simulink model "hdv_hydroelectropowertrain_model"  (R2023b)
settings: Solver=ode1be  StartTime=0.0  StopTime=simulation_length  FixedStep=tsample  MaxStep=tsample
values from neighbouring files (symbols this model uses):
  alpha = 35    [init_model.m]
  Apump = [0 1; 0 0]    [init_model.m]
  available_torque = torque_base+torque_friction_base    [init_model.m]
  Bpump = [0 1]'    [init_model.m]
  btheta_shaft = 2e2    (= 200)    [init_model.m]
  C1 = 10    [init_model.m]
  consumption = [consumption_1, consumption_2, consumption_3, consumption_4,          consumption_5, consumption_6, consumption_7, consumption_8,          consumption_9, consumption_10, consumption_11, consumption_12,          consumption_13, consumption_14, consumption_15, consumption_16          ]    [ic_engine_data.m]
  Cpump = [k 0]    [init_model.m]
  dp_lim = 400    [init_model.m]
  E0 = 3.685    [init_model.m]
  E1 = 0.2156    [init_model.m]
  E2 = 0    [init_model.m]
  E3 = 0    [init_model.m]
  E_1 = -1.031    [init_model.m]
  Elog = -0.05    [init_model.m]
  eta_v_m = 0.98    [init_model.m]
  eta_v_p = 0.97    [init_model.m]
  ki_dp_comp = 1/dp_lim    (= 0.0025)    [init_model.m]
  ki_te_comp = 2/te_lim    [init_model.m]
  kp_ctrl_m = 1    [init_model.m]
  kp_dp_comp = 0.5/dp_lim    (= 0.00125)    [init_model.m]
  kp_te_comp = 1/te_lim    [init_model.m]
  Kpump = acker(Apump,Bpump,poles)    [init_model.m]
  load_blade_enable = 0    [init_model.m]
  Lpump = acker(Apump',Cpump',pole_so)'    [init_model.m]
  M = 125    [init_model.m]
  Ncell = 185    [init_model.m]
  Npump = -1/(Cpump*inv(Apump-Bpump*Kpump)*Bpump)    [init_model.m]
  omega_e_rpm_ref = 1700    [init_model.m]
  omega_l_max_rpm = omega_l_max/(2*pi)*60    (= 50.3075969543)    [init_model.m]
  q1Kalman = tsample^2*1e-2    (= 1e-08)    [init_model.m]
  q2Kalman = tsample^1*1e-1    (= 0.0001)    [init_model.m]
  q3Kalman = 0    [init_model.m]
  Qhr = 400    [init_model.m]
  R0 = 0.015    [init_model.m]
  R1 = 0.015    [init_model.m]
  R_tg = 1.16/2    (= 0.58)    [init_model.m]
  rKalman = 1    [init_model.m]
  rpm_base = [620 700 800 900 1000 1100 1200 1300 1400 1500 1600 1700 1800      1900 2000 2100]    [ic_engine_data.m]
  rpm_consumption = rpm_base    [ic_engine_data.m]
  simulation_length = 245    [init_model.m]
  tau_load = 75e3    (= 75000)    [init_model.m]
  tau_load_max = 1600*41.4    (= 66240)    [init_model.m]
  Tc = tsample    (= 0.001)    [init_model.m]
  torque_base = [max(torque_16_data) max(torque_15_data) max(torque_14_data)      max(torque_13_data) max(torque_12_data) max(torque_11_data)      max(torque_10_data) max(torque_9_data) max(torque_8_data)      max(torque_7_data) max(torque_6_data) max(torque_5_data)      max(torque_4_data) max(torque_3_data) max(torque_2_data)      max(torque_1_data)]    [ic_engine_data.m]
  torque_consumption = torque_reference    [ic_engine_data.m]
  torque_friction_base = -(rpm_base./60*2*pi)*0.25-(rpm_base./60*2*pi).^2*5.2e-4    [ic_engine_data.m]
  tsample = 1e-3    (= 0.001)    [init_model.m]
  v_track1_ref = 8    [init_model.m]
  v_track2_ref = 8    [init_model.m]
  valve_mmorifice_max = 2.75    [init_model.m]
  xv_m_max = 1.2    [init_model.m]
undefined symbols (not defined in the file or in its folder): magnitude
libraries: fl_lib x381, nesl_utility x162, linear_swashplate_ctrl_lib x8, flexshaft_lib x5, bichamber_piston_lib x5, variable_displacement_motor_lib x4, variable_displacement_pump_lib x4, fixed_displacement_pump_lib x4, relief_valve_lib x4, inverse_shuttle_valve_lib x4, hydrostatic_threeway_valve_bichamber_piston_lib x4, hydrostatic_fourway_valve_bichamber_piston_lib x4
(part 3 of 9)

== system hdv_hydroelectropowertrain_model/PR776_powertrain/constant_pressure_source/Pressure controlled pump1 ==
  Hydraulic Flow Rate Sensor : fl_lib/Hydraulic/Hydraulic Sensors/Hydraulic Flow Rate Sensor
  Hydraulic Pressure Sensor : fl_lib/Hydraulic/Hydraulic Sensors/Hydraulic Pressure Sensor
  Hydraulic Reference : fl_lib/Hydraulic/Hydraulic Elements/Hydraulic Reference
  PS-Simulink Converter : nesl_utility/PS-Simulink Converter  PhysicalDomain=network_engine_domain  SubClassName=ps_output  LeftPortType=input  RightPortType=output  PseudoPeriodic=off  Frequencies=[]  VectorFormat=1-D array  Unit=bar  AffineConversion=on
  PS-Simulink Converter1 : nesl_utility/PS-Simulink Converter  PhysicalDomain=network_engine_domain  SubClassName=ps_output  LeftPortType=input  RightPortType=output  PseudoPeriodic=off  Frequencies=[]  VectorFormat=1-D array  Unit=l/min  AffineConversion=on
  PS-Simulink Converter{2..5} (4 alike) : nesl_utility/PS-Simulink Converter  PhysicalDomain=network_engine_domain  SubClassName=ps_output  LeftPortType=input  RightPortType=output  PseudoPeriodic=off  Frequencies=[]  VectorFormat=1-D array  Unit=1  AffineConversion=off
  Pressure controlled pump : pressure_controlled_pump_lib/Pressure controlled pump  Vd_nom=62.3*4 cm^3/rev  pnom=250 bar  b=0.1 N*m/(rad/s)  inertia_pump=0.027 kg*m^2  vd_lim_max=0.98  vd_lim_min=0  p_set=258 bar  p_reg=8 bar  x_rv_max=12 mm  kpc=2  kic=40 1/s  te_specify=off  te_priority=None  te=0 N*m  te_nominal_specify=off  te_nominal_unit=N*m  te_nominal_value=1  qA_specify=off  qA_priority=None  qA=0 m^3/s  qA_nominal_specify=off  qA_nominal_unit=m^3/s  qA_nominal_value=1  qB_specify=off  qB_priority=None  qB=0 m^3/s  qB_nominal_specify=off  qB_nominal_unit=m^3/s  qB_nominal_value=1  qd_specify=off  qd_priority=None  qd=0 m^3/s  qd_nominal_specify=off  qd_nominal_unit=m^3/s  qd_nominal_value=1  dp_specify=off  dp_priority=None  dp=0 Pa  dp_nominal_specify=off  dp_nominal_unit=Pa  dp_nominal_value=1  vd_specify=off  vd_priority=None  vd=0  vd_nominal_specify=off  vd_nominal_unit=1  vd_nominal_value=1  vd_i_specify=off  vd_i_priority=None  vd_i=0  vd_i_nominal_specify=off  vd_i_nominal_unit=1  vd_i_nominal_value=1  we_specify=off  we_priority=None  we=0 rad/s  we_nominal_specify=off  we_nominal_unit=rad/s  we_nominal_value=1
      settings: InternalSimscapePortConfiguration="{\"Bottom\":[],\"Left\":[{\"id\":\"cW\",\"label\":\"cW\",\"type\":\"foundation.mechanical.rotational.rotational\"},{\"id\":\"dp_ref\",\"label\":\"Pressure set-point\",\"type\":\"input\"}],\"Right\":[{\"id\":\"cA\",\"label\":\"cA\",\"type\":\"foundation.hydraulic.hydraulic\"},{\"id\":\"cB\",\"label\":\"cB\",\"type\":\"foundation.hydraulic.hydraulic\"},{\"id\":\"qleak\",\"label\":\"qleak\",\"type\":\"output\"},{\"id\":\"taup\",\"label\":\"taup\",\"type\":\"output\"},{\"id\":\"vdi\",\"label\":\"vdi\",\"type\":\"output\"},{\"id\":\"pflow\",\"label\":\"pflow\",\"type\":\"output\"}],\"Top\":[]}"
  flow : Scope
  leak/ptorque : Scope  NumInputPorts=3
  pressure : Scope
  pump_flow : Scope
  pS : PMIOPort  Side=Right
  shaft : PMIOPort  Port=2  Side=Left
  pT : PMIOPort  Port=3  Side=Right
  wires:
  PS-Simulink Converter1/1 -> flow/1
  PS-Simulink Converter4/1 -> leak/ptorque/3  "vd"
  PS-Simulink Converter3/1 -> leak/ptorque/2  "torque"
  PS-Simulink Converter5/1 -> pump_flow/1
  PS-Simulink Converter2/1 -> leak/ptorque/1  "leak"
  PS-Simulink Converter/1 -> pressure/1
  connections:
  shaft/RConn1 -- Pressure controlled pump/LConn1
  Pressure controlled pump/RConn4 -- PS-Simulink Converter3/LConn1
  Pressure controlled pump/RConn3 -- PS-Simulink Converter2/LConn1
  Hydraulic Flow Rate Sensor/RConn1 -- PS-Simulink Converter1/LConn1
  Hydraulic Pressure Sensor/LConn1 -- pS/RConn1 -- Hydraulic Flow Rate Sensor/RConn2
  Hydraulic Reference/LConn1 -- Pressure controlled pump/RConn2 -- pT/RConn1 -- Hydraulic Pressure Sensor/RConn1
  Pressure controlled pump/RConn1 -- Hydraulic Flow Rate Sensor/LConn1
  Pressure controlled pump/RConn5 -- PS-Simulink Converter4/LConn1
  Pressure controlled pump/RConn6 -- PS-Simulink Converter5/LConn1
  PS-Simulink Converter/LConn1 -- Hydraulic Pressure Sensor/RConn2

== system hdv_hydroelectropowertrain_model/PR776_powertrain/electrical_main_drive_train/LithiumIonBattery ==
  Bus Creator : BusCreator  Inputs=4
  Current Sensor : fl_lib/Electrical/Electrical Sensors/Current Sensor
  Current Sensor1 : fl_lib/Electrical/Electrical Sensors/Current Sensor
  Electrical Reference1 : fl_lib/Electrical/Electrical Elements/Electrical Reference
  PS-Simulink Converter1 : nesl_utility/PS-Simulink Converter  PhysicalDomain=network_engine_domain  SubClassName=ps_output  LeftPortType=input  RightPortType=output  PseudoPeriodic=off  Frequencies=[]  VectorFormat=1-D array  Unit=1  AffineConversion=off
  PS-Simulink Converter4 : nesl_utility/PS-Simulink Converter  PhysicalDomain=network_engine_domain  SubClassName=ps_output  LeftPortType=input  RightPortType=output  PseudoPeriodic=off  Frequencies=[]  VectorFormat=1-D array  Unit=1  AffineConversion=off
  PS-Simulink Converter5 : nesl_utility/PS-Simulink Converter  PhysicalDomain=network_engine_domain  SubClassName=ps_output  LeftPortType=input  RightPortType=output  PseudoPeriodic=off  Frequencies=[]  VectorFormat=1-D array  Unit=V  AffineConversion=on
  Resistor1 : fl_lib/Electrical/Electrical Elements/Resistor  R=1e4 Ohm  i_specify=off  i_priority=None  i=0 A  i_nominal_specify=off  i_nominal_unit=A  i_nominal_value=1  v_specify=off  v_priority=None  v=0 V  v_nominal_specify=off  v_nominal_unit=V  v_nominal_value=1
  Resistor2 : fl_lib/Electrical/Electrical Elements/Resistor  R=1e4 Ohm  i_specify=off  i_priority=None  i=0 A  i_nominal_specify=off  i_nominal_unit=A  i_nominal_value=1  v_specify=off  v_priority=None  v=0 V  v_nominal_specify=off  v_nominal_unit=V  v_nominal_value=1
  Unit Delay5 : UnitDelay  SampleTime=tsample  HasFrameUpgradeWarning=on
  Voltage Sensor : fl_lib/Electrical/Electrical Sensors/Voltage Sensor
  lithium ion cell analytical ocv : Subsystem
  Uout+ : PMIOPort  Side=Right
  Uout- : PMIOPort  Port=2  Side=Right
  Uin+ : PMIOPort  Port=3  Side=Left
  Uin- : PMIOPort  Port=4  Side=Left
  lithiumIonBattery_Data : Outport
  tag scope: vout_battery=global
  wires:
  PS-Simulink Converter5/1 -> Unit Delay5/1
  PS-Simulink Converter4/1 -> [iout_battery]  "i batt"
  Unit Delay5/1 -> [vout_battery]
  Bus Creator/1 -> lithiumIonBattery_Data/1
  [iout_battery] -> Bus Creator/1  "Iout_battery"
  [vout_battery] -> Bus Creator/2  "Vout_battery"
  [soc_battery] -> Bus Creator/3  "soc_battery"
  PS-Simulink Converter1/1 -> [iin_battery]  "i batt"
  [iin_battery] -> Bus Creator/4  "iin_battery"
  connections:
  Current Sensor/RConn1 -- PS-Simulink Converter4/LConn1
  Current Sensor/RConn2 -- Voltage Sensor/LConn1 -- Resistor2/LConn1 -- Uout+/RConn1
  Voltage Sensor/RConn1 -- PS-Simulink Converter5/LConn1
  Voltage Sensor/RConn2 -- Resistor1/RConn1 -- Uin-/RConn1 -- Electrical Reference1/LConn1 -- lithium ion cell analytical ocv/RConn2 -- Resistor2/RConn1 -- Uout-/RConn1
  lithium ion cell analytical ocv/RConn1 -- Current Sensor1/RConn2 -- Current Sensor/LConn1
  Current Sensor1/RConn1 -- PS-Simulink Converter1/LConn1
  Uin+/RConn1 -- Resistor1/LConn1 -- Current Sensor1/LConn1

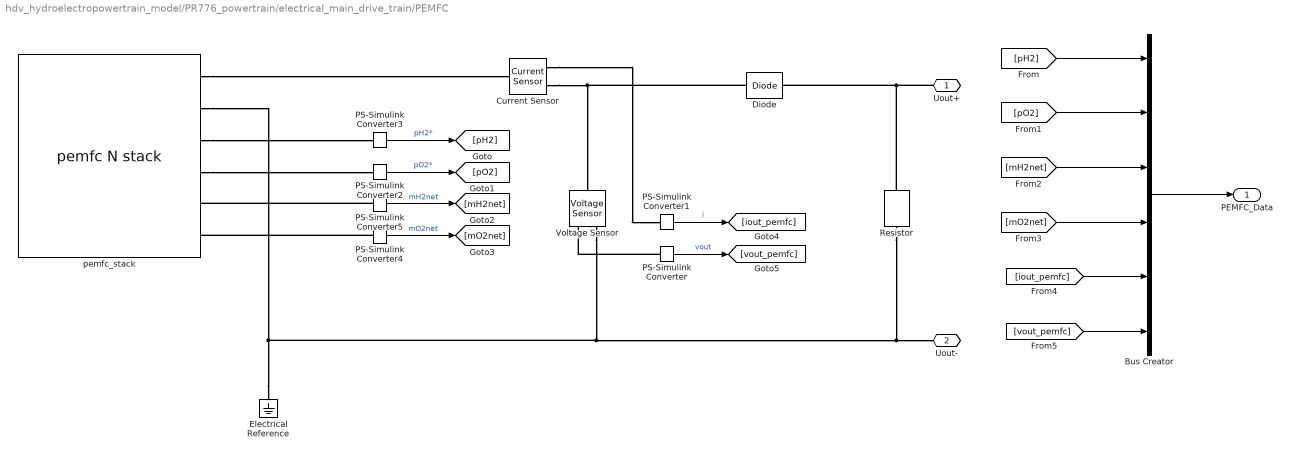
== system hdv_hydroelectropowertrain_model/PR776_powertrain/electrical_main_drive_train/PEMFC ==
  Bus Creator : BusCreator  Inputs=6
  Current Sensor : fl_lib/Electrical/Electrical Sensors/Current Sensor
  Diode : ee_lib/Semiconductors & Converters/Diode  ModelType=ee.enum.diode.modelType.pwl  TableType=ee.enum.diode.tableType.IfMat  IfMat=[.07, .12, .19, 1.75, 4.24, 7.32, 11.2; .16, .3, .72, 2.14, 5.02, 8.35, 13.12] A  VfMat=[.9, 1.15, 1.25, 1.5, 1.75, 2.17, 2.6, 2.85; .58, .68, .75, 1.1, 1.38, 1.77, 2.27, 2.7] V  TjVec=[25, 125] degC  VfVec=[.5, .7, .9, 1.3, 1.7, 2.1, 2.5] V  IfVec=[.1, .2, .5, 1, 2, 4, 7, 10] A  Vf=0.6 V  Ron=0.3 Ohm  Goff=1e-8 S  prmExp=ee.enum.diode.expParam.useTwo  I12=[.0137, .545] A  V12=[.6, .7] V  RS=0 Ohm  Tmeas=25 degC  IS=1e-12 A  ec=1  I1=0.0137 A  V1=0.6 V  N_series=1  N_parallel=1  ZenerEnable=false  Rz=0.3 Ohm  BV=inf V  C_param=ee.enum.diode.capParam.fixed  CJ=5 pF  CJ0=5 pF  Vvec=[.1, 10, 100] V  Cvec=[3.5, 1, .4] pF  VJ=1 V  Mgrad=0.5  FC=0.5  Q_param=ee.enum.diode.recoveryParam.off  iRM=-7.15 A  iF=4 A  didt=-750 A/us  trr_factor=3  trr=115 ns  Qrr=1500 s*uA  Vr=-600 V  Ls=150 nH  Erec=0.03 J  TT=50 ns  tau=100 ns  T_param=ee.enum.diode.temperatureParam.off  Tdevice=25 degC  I1_T2=0.245 A  V1_T2=0.5 V  IS_T2=1.25e-7 A  Tmeas2=125 degC  XTI_param=ee.enum.diode.xtiParam.pn  XTI=3  EG_param=ee.enum.diode.egapParam.material_si  EG=1.11 eV  dBVdT=0 V/K  enable_faults=ee.enum.enable.no  fault_action=simscape.enum.assert.action.none  fault_types=ee.enum.diode.faults.open  tau_fault=1e-3 s  IfMat_faulted=[.07, .12, .19, 1.75, 4.24, 7.32, 11.2; .16, .3, .72, 2.14, 4.02, 6.35, 9.12] A  VfMat_faulted=[.9, 1.15, 1.25, 1.5, 1.75, 2.17, 2.6, 2.85; .58, .68, .75, 1.1, 1.38, 1.77, 2.27, 2.7] V  VfVec_faulted=[.5, .7, .9, 1.3, 1.7, 2.1, 2.5] V  IfVec_faulted=[.1, .2, .5, 1, 2, 4, 7, 10] A  Ropen_faulted=1000 Ohm  Gshort_faulted=1000 1/Ohm  Vf_faulted=0.6 V  Ron_faulted=0.3 Ohm  Goff_faulted=1e-8 S  I12_faulted=[.0137, .545] A  V12_faulted=[.6, .7] V  IS_faulted=1e-12 A  ec_faulted=1  I1_faulted=0.0137 A  V1_faulted=0.6 V  RS_faulted=0 Ohm  Rz_faulted=0.3 Ohm  BV_faulted=inf V  Cscale_faulted=100  fault_trigger=ee.enum.faults.faultTrigger.temporal  t_fault=inf s  max_permissible_voltage=inf V  n_fail_on_voltage=1  max_permissible_current=inf A  t_fail_on_current=1 s  max_permissible_dVdt=inf V/s  enable_fault_input=simscape.enum.onoff.off  i_specify=off  i_priority=None  i=0 A  i_nominal_specify=off  i_nominal_unit=A  i_nominal_value=1  v_specify=off  v_priority=None  v=0 V  v_nominal_specify=off  v_nominal_unit=V  v_nominal_value=1  v_capacitor_specify=off  v_capacitor_priority=None  v_capacitor=0 V  v_capacitor_nominal_specify=off  v_capacitor_nominal_unit=V  v_capacitor_nominal_value=1  faulted_specify=off  faulted_priority=None  faulted=0  faulted_nominal_specify=off  faulted_nominal_unit=1  faulted_nominal_value=1  i_diode_specify=off  i_diode_priority=None  i_diode=0 A  i_diode_nominal_specify=off  i_diode_nominal_unit=A  i_diode_nominal_value=1  v_diode_specify=off  v_diode_priority=None  v_diode=0 V  v_diode_nominal_specify=off  v_diode_nominal_unit=V  v_diode_nominal_value=1  i_capacitor_specify=off  i_capacitor_priority=None  i_capacitor=0 A  i_capacitor_nominal_specify=off  i_capacitor_nominal_unit=A  i_capacitor_nominal_value=1  power_dissipated_specify=off  power_dissipated_priority=None  power_dissipated=0 W  power_dissipated_nominal_specify=off  power_dissipated_nominal_unit=W  power_dissipated_nominal_value=1  fidelity_level=ee.enum.diode.fidelity.includeChargeDyn  rec_loss_model=ee.enum.diode.reverseRecoveryModel.fixed  ErecVal=0 J  scaleWithIandV=true  ErecMat=zeros(2, 3) J  TjrecVec=[298.15, 398.15] K  IfrecVec=[.1, 1, 10] A  IrecVal=10 A  VrecVal=10 V  tFilter=1 / 1000 / 100 s  max_permissible_temperature=inf K  t_fail_on_temperature=1 s  thermal_network_parameterization=ee.enum.thermalNetworkTopology.junctionCase  Rth=[0, 10] K/W  Rth_Cauer=[1, 3, 10] K/W  Rth_Foster=[4, 6] K/W  thermal_mass_parameterization=ee.enum.thermalNetwork.timeconstant  thermal_mass=[0, 1] J/K  thermal_mass_Cauer=[.1, .3, 1] J/K  thermal_mass_Foster=[1.5, 3] J/K  thermal_time_constant=[0, 10] s  thermal_time_constant_Cauer=[1, 3, 10] s  thermal_time_constant_Foster=[6, 18] s  thermal_mass_initial_temperatures=[25, 25] degC  thermal_mass_initial_temperatures_Cauer=[25, 25, 25] degC  junction_thermal_mass=0.01 J/K  Tvec_initial_Foster=[25, 25, 25, 25] degC  no_thermal_network=0  junction_temperature_specify=off  junction_temperature_priority=None  junction_temperature=25 degC  junction_temperature_nominal_specify=off  junction_temperature_nominal_unit=degC  junction_temperature_nominal_value=1
  Electrical Reference : fl_lib/Electrical/Electrical Elements/Electrical Reference
  PS-Simulink Converter{,1..5} (6 alike) : nesl_utility/PS-Simulink Converter  PhysicalDomain=network_engine_domain  SubClassName=ps_output  LeftPortType=input  RightPortType=output  PseudoPeriodic=off  Frequencies=[]  VectorFormat=1-D array  Unit=inherit  AffineConversion=off
  Resistor : fl_lib/Electrical/Electrical Elements/Resistor  R=1e2 Ohm  i_specify=off  i_priority=None  i=0 A  i_nominal_specify=off  i_nominal_unit=A  i_nominal_value=1  v_specify=off  v_priority=None  v=0 V  v_nominal_specify=off  v_nominal_unit=V  v_nominal_value=1
  Voltage Sensor : fl_lib/Electrical/Electrical Sensors/Voltage Sensor
  pemfc_stack : pemfc_stack_lib/pemfc N stack  F=96487 s*A/mol  R=8.314 J/K/mol  T=298 K  DGibbs=285800 J/mol  n=2  Va=Va m^3  Vc=Vc m^3  tau_a=0.15 s  tau_c=0.15 s  p0=1e5 Pa  Ncells=Ncells  Rohm0=Rohm0 Ohm  Ract=Ract Ohm  Rconc=Rconc Ohm  Cdlc=Cdlc F  e_specify=off  e_priority=None  e=0 V  e_nominal_specify=off  e_nominal_unit=V  e_nominal_value=1  u_specify=off  u_priority=None  u=0 V  u_nominal_specify=off  u_nominal_unit=V  u_nominal_value=1  uc_specify=off  uc_priority=None  uc=0 V  uc_nominal_specify=off  uc_nominal_unit=V  uc_nominal_value=1  icell_specify=off  icell_priority=None  icell=0 A  icell_nominal_specify=off  icell_nominal_unit=A  icell_nominal_value=1  pH2_star_specify=off  pH2_star_priority=High  pH2_star=3  pH2_star_nominal_specify=off  pH2_star_nominal_unit=1  pH2_star_nominal_value=1  pO2_star_specify=off  pO2_star_priority=High  pO2_star=3  pO2_star_nominal_specify=off  pO2_star_nominal_unit=1  pO2_star_nominal_value=1  mH2_net_specify=off  mH2_net_priority=None  mH2_net=0 mol/s  mH2_net_nominal_specify=off  mH2_net_nominal_unit=mol/s  mH2_net_nominal_value=1  mO2_net_specify=off  mO2_net_priority=None  mO2_net=0 mol/s  mO2_net_nominal_specify=off  mO2_net_nominal_unit=mol/s  mO2_net_nominal_value=1  mask(pemfc N stack){}
      settings: InternalSimscapePortConfiguration="{\"Bottom\":[],\"Left\":[],\"Right\":[{\"id\":\"u_p\",\"label\":\"u+\",\"type\":\"foundation.electrical.electrical\"},{\"id\":\"u_n\",\"label\":\"u-\",\"type\":\"foundation.electrical.electrical\"},{\"id\":\"pH2_out\",\"label\":\"pH2*\",\"type\":\"output\"},{\"id\":\"pO2_out\",\"label\":\"pO2*\",\"type\":\"output\"},{\"id\":\"mH2_net_out\",\"label\":\"mH2net\",\"type\":\"output\"},{\"id\":\"mO2_net_out\",\"label\":\"mO2net\",\"type\":\"output\"}],\"Top\":[]}"
  Uout+ : PMIOPort  Side=Right
  Uout- : PMIOPort  Port=2  Side=Right
  PEMFC_Data : Outport
  wires:
  PS-Simulink Converter2/1 -> [pO2]  "pO2*"
  PS-Simulink Converter1/1 -> [iout_pemfc]  "i"
  PS-Simulink Converter/1 -> [vout_pemfc]  "vout"
  PS-Simulink Converter3/1 -> [pH2]  "pH2*"
  PS-Simulink Converter5/1 -> [mH2net]  "mH2net"
  PS-Simulink Converter4/1 -> [mO2net]  "mO2net"
  Bus Creator/1 -> PEMFC_Data/1
  [pH2] -> Bus Creator/1
  [vout_pemfc] -> Bus Creator/6
  [pO2] -> Bus Creator/2
  [mH2net] -> Bus Creator/3
  [mO2net] -> Bus Creator/4
  [iout_pemfc] -> Bus Creator/5
  connections:
  pemfc_stack/RConn3 -- PS-Simulink Converter3/LConn1
  PS-Simulink Converter/LConn1 -- Voltage Sensor/RConn1
  pemfc_stack/RConn1 -- Current Sensor/LConn1
  pemfc_stack/RConn4 -- PS-Simulink Converter2/LConn1
  Electrical Reference/LConn1 -- Voltage Sensor/RConn2 -- Resistor/RConn1 -- Uout-/RConn1 -- pemfc_stack/RConn2
  Current Sensor/RConn1 -- PS-Simulink Converter1/LConn1
  PS-Simulink Converter4/LConn1 -- pemfc_stack/RConn6
  PS-Simulink Converter5/LConn1 -- pemfc_stack/RConn5
  Current Sensor/RConn2 -- Diode/LConn1 -- Voltage Sensor/LConn1
  Resistor/LConn1 -- Uout+/RConn1 -- Diode/RConn1

== system hdv_hydroelectropowertrain_model/PR776_powertrain/electrical_main_drive_train/battery_management ==
  vout(k) : Inport
  i(k) : Inport  Port=2
  Constant : Constant  Value=tsample
  Constant1 : Constant  Value=Qhr
  Constant2 : Constant  Value=q1Kalman
  Constant3 : Constant  Value=q2Kalman
  Constant4 : Constant  Value=q3Kalman
  Constant5 : Constant  Value=rKalman
  Constant6 : Constant  Value=tsample
  Constant7 : Constant  Value=Qhr
  Selector : Selector  InputPortWidth=3  IndexOptions=Index vector (dialog)  Indices=1  OutputSizes=1
  Unit Delay4 : UnitDelay  SampleTime=tsample  HasFrameUpgradeWarning=on
  kalman_observer_gains : MATLAB Function  TreatAsAtomicUnit=on  SystemSampleTime=tsample
  lithium-ion battery model : MATLAB Function  TreatAsAtomicUnit=on  SystemSampleTime=tsample
  SOC(k) : Outport
  vout_hat : Outport  Port=2
  wires:
  lithium-ion battery model/1(SOC) -> SOC(k)/1  "SOC"
  Constant6/1 -> kalman_observer_gains/2(ts)
  vout(k)/1 -> lithium-ion battery model/7(vout)
  kalman_observer_gains/2(l2) -> lithium-ion battery model/5(l2)
  Selector/1 -> Unit Delay4/1
  kalman_observer_gains/3(l3) -> lithium-ion battery model/6(l3)
  kalman_observer_gains/1(l1) -> lithium-ion battery model/4(l1)
  Constant7/1 -> kalman_observer_gains/8(Qhr)
  Constant1/1 -> lithium-ion battery model/3(Qhr)
  Constant5/1 -> kalman_observer_gains/7(r)
  Constant4/1 -> kalman_observer_gains/6(q3)
  Constant2/1 -> kalman_observer_gains/4(q1)
  Constant/1 -> lithium-ion battery model/2(ts)
  i(k)/1 -> kalman_observer_gains/1(iz), lithium-ion battery model/1(iz)
  lithium-ion battery model/3(x) -> Selector/1  "x(k+1|k)"
  Unit Delay4/1 -> kalman_observer_gains/3(z)  "x(k|k-1)"
  Constant3/1 -> kalman_observer_gains/5(q2)
  lithium-ion battery model/2(u) -> vout_hat/1  "vout_hat"

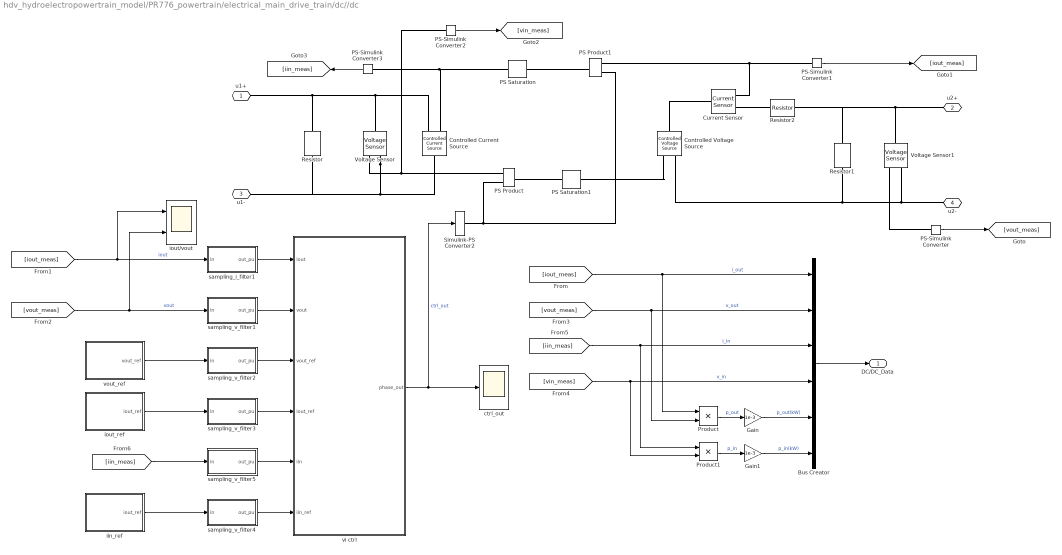
== system hdv_hydroelectropowertrain_model/PR776_powertrain/electrical_main_drive_train/dc//dc ==
  Bus Creator : BusCreator  Inputs=6
  Controlled Current Source : fl_lib/Electrical/Electrical Sources/Controlled Current Source
  Controlled Voltage Source : fl_lib/Electrical/Electrical Sources/Controlled Voltage Source
  Current Sensor : fl_lib/Electrical/Electrical Sensors/Current Sensor
  Gain : Gain  Gain=1e-3
  Gain1 : Gain  Gain=1e-3
  PS Product : fl_lib/Physical Signals/Functions/PS Product
  PS Product1 : fl_lib/Physical Signals/Functions/PS Product
  PS Saturation : fl_lib/Physical Signals/Nonlinear Operators/PS Saturation  upper_limit=inf A  lower_limit=-inf A
  PS Saturation1 : fl_lib/Physical Signals/Nonlinear Operators/PS Saturation  upper_limit=inf V  lower_limit=-inf V
  PS-Simulink Converter : nesl_utility/PS-Simulink Converter  PhysicalDomain=network_engine_domain  SubClassName=ps_output  LeftPortType=input  RightPortType=output  PseudoPeriodic=off  Frequencies=[]  VectorFormat=1-D array  Unit=inherit  AffineConversion=off
  PS-Simulink Converter1 : nesl_utility/PS-Simulink Converter  PhysicalDomain=network_engine_domain  SubClassName=ps_output  LeftPortType=input  RightPortType=output  PseudoPeriodic=off  Frequencies=[]  VectorFormat=1-D array  Unit=inherit  AffineConversion=on
  PS-Simulink Converter2 : nesl_utility/PS-Simulink Converter  PhysicalDomain=network_engine_domain  SubClassName=ps_output  LeftPortType=input  RightPortType=output  PseudoPeriodic=off  Frequencies=[]  VectorFormat=1-D array  Unit=inherit  AffineConversion=off
  PS-Simulink Converter3 : nesl_utility/PS-Simulink Converter  PhysicalDomain=network_engine_domain  SubClassName=ps_output  LeftPortType=input  RightPortType=output  PseudoPeriodic=off  Frequencies=[]  VectorFormat=1-D array  Unit=inherit  AffineConversion=off
  Product : Product
  Product1 : Product
  Resistor : fl_lib/Electrical/Electrical Elements/Resistor  R=1e4 Ohm  i_specify=off  i_priority=None  i=0 A  i_nominal_specify=off  i_nominal_unit=A  i_nominal_value=1  v_specify=off  v_priority=None  v=0 V  v_nominal_specify=off  v_nominal_unit=V  v_nominal_value=1
  Resistor1 : fl_lib/Electrical/Electrical Elements/Resistor  R=1e4 Ohm  i_specify=off  i_priority=None  i=0 A  i_nominal_specify=off  i_nominal_unit=A  i_nominal_value=1  v_specify=off  v_priority=None  v=0 V  v_nominal_specify=off  v_nominal_unit=V  v_nominal_value=1
  Resistor2 : fl_lib/Electrical/Electrical Elements/Resistor  R=5e-3 Ohm  i_specify=off  i_priority=None  i=0 A  i_nominal_specify=off  i_nominal_unit=A  i_nominal_value=1  v_specify=off  v_priority=None  v=0 V  v_nominal_specify=off  v_nominal_unit=V  v_nominal_value=1
  Simulink-PS Converter2 : nesl_utility/Simulink-PS Converter  PhysicalDomain=network_engine_domain  SubClassName=ps_input  LeftPortType=input  RightPortType=output  PseudoPeriodic=off  Frequencies=[]  NoiseDistribution=none  NoiseParameters=[]  Unit=1  AffineConversion=on  FilteringAndDerivatives=zero  SimscapeFilterOrder=2  InputFilterTimeConstant=tsample  UdotUserProvided=2
  Voltage Sensor : fl_lib/Electrical/Electrical Sensors/Voltage Sensor
  Voltage Sensor1 : fl_lib/Electrical/Electrical Sensors/Voltage Sensor
  ctrl_out : Scope
  iin_ref : Subsystem
  iout/vout : Scope  NumInputPorts=2
  iout_ref : Subsystem
  sampling_i_filter1 : Subsystem
  sampling_v_filter1 : Subsystem
  sampling_v_filter2 : Subsystem
  sampling_v_filter3 : Subsystem
  sampling_v_filter4 : Subsystem
  sampling_v_filter5 : Subsystem
  vi ctrl : Subsystem
  vout_ref : Subsystem
  u1+ : PMIOPort  Side=Left
  u2+ : PMIOPort  Port=2  Side=Right
  u1- : PMIOPort  Port=3  Side=Left
  u2- : PMIOPort  Port=4  Side=Right
  DC/DC_Data : Outport
  wires:
  vi ctrl/1(phase_out) -> Simulink-PS Converter2/1, ctrl_out/1  "ctrl_out"
  [iout_meas] -> iout/vout/1, sampling_i_filter1/1(in)  "iout"
  sampling_v_filter1/1(out_pu) -> vi ctrl/2(vout)
  sampling_v_filter2/1(out_pu) -> vi ctrl/3(vout_ref)
  [vout_meas] -> iout/vout/2, sampling_v_filter1/1(in)  "vout"
  sampling_i_filter1/1(out_pu) -> vi ctrl/1(iout)
  vout_ref/1(vout_ref) -> sampling_v_filter2/1(in)
  PS-Simulink Converter/1 -> [vout_meas]
  iout_ref/1(iout_ref) -> sampling_v_filter3/1(in)
  sampling_v_filter3/1(out_pu) -> vi ctrl/4(iout_ref)
  Bus Creator/1 -> DC/DC_Data/1
  [iout_meas] -> Product/1, Bus Creator/1  "i_out"
  [vout_meas] -> Product/2, Bus Creator/2  "v_out"
  PS-Simulink Converter2/1 -> [vin_meas]
  [vin_meas] -> Product1/2, Bus Creator/4  "v_in"
  PS-Simulink Converter3/1 -> [iin_meas]
  [iin_meas] -> Product1/1, Bus Creator/3  "i_in"
  Product/1 -> Gain/1  "p_out"
  Product1/1 -> Gain1/1  "p_in"
  Gain/1 -> Bus Creator/5  "p_out(kW)"
  Gain1/1 -> Bus Creator/6  "p_in(kW)"
  PS-Simulink Converter1/1 -> [iout_meas]
  iin_ref/1(iout_ref) -> sampling_v_filter4/1(in)
  sampling_v_filter4/1(out_pu) -> vi ctrl/6(iin_ref)
  sampling_v_filter5/1(out_pu) -> vi ctrl/5(iin)
  [iin_meas] -> sampling_v_filter5/1(in)
  connections:
  Simulink-PS Converter2/RConn1 -- PS Product/LConn2 -- PS Product1/LConn1
  Current Sensor/RConn1 -- PS-Simulink Converter1/LConn1 -- PS Product1/LConn2
  Voltage Sensor/RConn1 -- PS-Simulink Converter2/LConn1 -- PS Product/LConn1
  Voltage Sensor/RConn2 -- Resistor/RConn1 -- u1-/RConn1 -- Controlled Current Source/LConn1
  Controlled Voltage Source/RConn2 -- Resistor1/RConn1 -- Voltage Sensor1/RConn2 -- u2-/RConn1
  Controlled Voltage Source/LConn1 -- Current Sensor/LConn1
  PS Product1/RConn1 -- PS Saturation/LConn1
  PS Product/RConn1 -- PS Saturation1/LConn1
  Voltage Sensor1/RConn1 -- PS-Simulink Converter/LConn1
  PS Saturation/RConn1 -- PS-Simulink Converter3/LConn1 -- Controlled Current Source/RConn1
  PS Saturation1/RConn1 -- Controlled Voltage Source/RConn1
  Voltage Sensor1/LConn1 -- Resistor2/RConn1 -- Resistor1/LConn1 -- u2+/RConn1
  Resistor/LConn1 -- Voltage Sensor/LConn1 -- Controlled Current Source/RConn2 -- u1+/RConn1
  Resistor2/LConn1 -- Current Sensor/RConn2

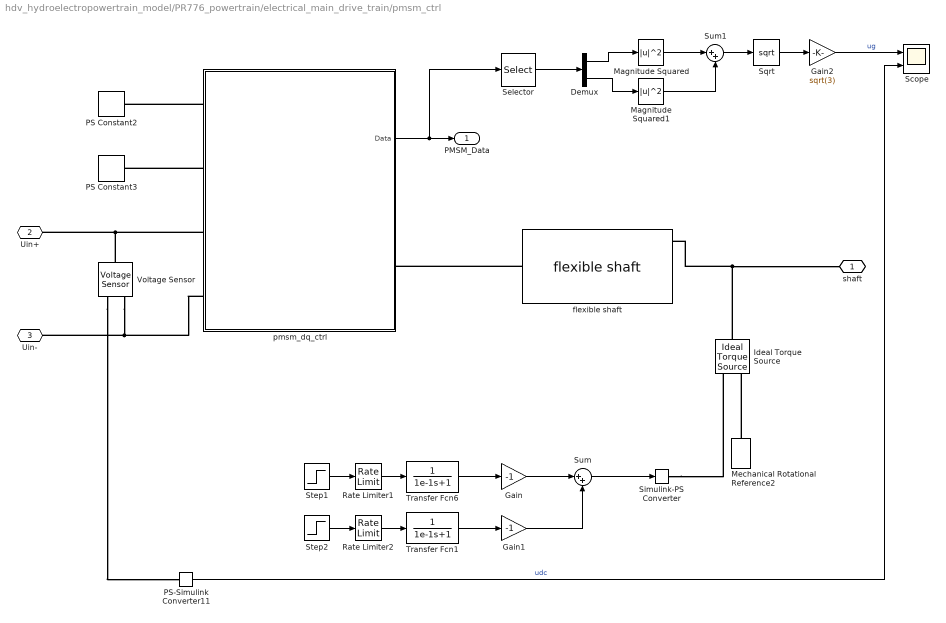
== system hdv_hydroelectropowertrain_model/PR776_powertrain/electrical_main_drive_train/pmsm_ctrl ==
  Demux : Demux  Outputs=2
  Gain : Gain  Gain=-1
  Gain1 : Gain  Gain=-1
  Gain2 : Gain  Gain=sqrt(3)
  Ideal Torque Source : fl_lib/Mechanical/Mechanical Sources/Ideal Torque Source
  Magnitude Squared : Math  Operator=magnitude^2
  Magnitude Squared1 : Math  Operator=magnitude^2
  Mechanical Rotational Reference2 : fl_lib/Mechanical/Rotational Elements/Mechanical Rotational Reference
  PS Constant2 : fl_lib/Physical Signals/Sources/PS Constant  constant=1800 rpm
  PS Constant3 : fl_lib/Physical Signals/Sources/PS Constant  constant=1140 N*m
  PS-Simulink Converter11 : nesl_utility/PS-Simulink Converter  PhysicalDomain=network_engine_domain  SubClassName=ps_output  LeftPortType=input  RightPortType=output  PseudoPeriodic=off  Frequencies=[]  VectorFormat=1-D array  Unit=V  AffineConversion=on
  Rate Limiter1 : RateLimiter  RisingSlewLimit=500  FallingSlewLimit=-500  SampleTimeMode=inherited
  Rate Limiter2 : RateLimiter  RisingSlewLimit=500  FallingSlewLimit=-500  SampleTimeMode=inherited
  Scope : Scope  NumInputPorts=2
  Selector : Selector  InputPortWidth=13  IndexOptions=Index vector (dialog)  Indices=[11 12]  OutputSizes=1
  Simulink-PS Converter : nesl_utility/Simulink-PS Converter  PhysicalDomain=network_engine_domain  SubClassName=ps_input  LeftPortType=input  RightPortType=output  PseudoPeriodic=off  Frequencies=[]  NoiseDistribution=none  NoiseParameters=[]  Unit=N*m  AffineConversion=on  FilteringAndDerivatives=provide  SimscapeFilterOrder=1  InputFilterTimeConstant=0.001  UdotUserProvided=0
  Sqrt : Sqrt
  Step1 : Step  Time=simulation_length/5  After=1140/20  SampleTime=0
  Step2 : Step  Time=simulation_length*2/5  After=1140/20  SampleTime=0
  Sum : Sum  Inputs=|++
  Sum1 : Sum  Inputs=|++
  Transfer Fcn1 : TransferFcn  Denominator=[1e-1 1]
  Transfer Fcn6 : TransferFcn  Denominator=[1e-1 1]
  Voltage Sensor : fl_lib/Electrical/Electrical Sensors/Voltage Sensor
  flexible shaft : flexshaft_lib/flexible shaft  b1=1e-2 N*m/(rad/s)  J1=1.25/5 kg*m^2  b2=1e-2 N*m/(rad/s)  J2=1.25/5 kg*m^2  b_theta=1 N*m/(rad/s)  k_theta=1e5 N*m/rad  w_1_specify=off  w_1_priority=None  w_1=0 rad/s  w_1_nominal_specify=off  w_1_nominal_unit=rad/s  w_1_nominal_value=1  w_2_specify=off  w_2_priority=None  w_2=0 rad/s  w_2_nominal_specify=off  w_2_nominal_unit=rad/s  w_2_nominal_value=1  t_1_specify=off  t_1_priority=None  t_1=0 N*m  t_1_nominal_specify=off  t_1_nominal_unit=N*m  t_1_nominal_value=1  t_2_specify=off  t_2_priority=None  t_2=0 N*m  t_2_nominal_specify=off  t_2_nominal_unit=N*m  t_2_nominal_value=1  t_theta_specify=off  t_theta_priority=None  t_theta=0 N*m  t_theta_nominal_specify=off  t_theta_nominal_unit=N*m  t_theta_nominal_value=1
      settings: InternalSimscapePortConfiguration="{\"Bottom\":[],\"Left\":[{\"id\":\"S1\",\"label\":\"S1\",\"type\":\"foundation.mechanical.rotational.rotational\"}],\"Right\":[{\"id\":\"S2\",\"label\":\"S2\",\"type\":\"foundation.mechanical.rotational.rotational\"},{\"id\":\"tau2\",\"label\":\"tau2\",\"type\":\"output\"},{\"id\":\"w2\",\"label\":\"w2\",\"type\":\"output\"}],\"Top\":[]}"
  pmsm_dq_ctrl : Subsystem  mask{control_mode=Speed Mode, torque_limitation=Torque limited from torque ref, polepairs=8, poles_unit=1, omega_m_max=2700, omega_m_max_unit=rpm, omega_m_nom=1800, omega_m_nom_unit=rpm, tau_nom=1140, tau_nom_unit=N*m, Rs=0.016, Rs_unit=Ohm, Ld=0.000274, Ld_unit=H, Lq=0.000263, Lq_unit=H, Ke=0.206, Ke_unit=V*s, Kt=3.35, Kt_unit=N*m/Arms, J=0.2, J_unit=kg*m^2, b=0.02, b_unit=N*m/(rad/s), kp_w=4, ki_w=35, kp_i=0.5, ki_i=18, kp_fw=0.1, ki_fw=2}
      mask prompts: control_mode "Enable Speed Mode"; torque_limitation "Enable Torque Limitation"; polepairs "Number of motor pole pairs"; omega_m_max "Maximum Speed"; omega_m_nom "Nominal Speed"; tau_nom "Nominal Torque"; Ke "Voltage Constant"; Kt "Torque Constant"; J "Rotor Inertia"; b "Viscosity"; kp_w "Proportional Speed Ctrl Gain"; ki_w "Integral Speed Ctrl Gain"; kp_i "Proportional Current Ctrl Gain"; ki_i "Integral Current Ctrl Gain"; kp_fw "Proportional Field Weakening Ctrl Gain"; ki_fw "Integral Field Weakening Ctrl Gain"
      mask init:
      | cm = get_param(gcb,'control_mode');
      | tl = get_param(gcb,'torque_limitation');
      | 
      | poles = 2*polepairs;
      | if Ke > 0
      |     phi_m = Ke;
      | elseif Kt > 0
      |     phi_m = Kt*sqrt(2)/3/polepairs;
      | else
      |     phi_m = 1;
      | end
      | 
      | omega_bez = omega_m_nom*polepairs/60*2*pi;
      | ubez = phi_m*omega_bez;
      | 
      | if Kt > 0
      |     ibez = tau_nom/Kt*sqrt(2);
      | else
      |     ibez = 2*tau_nom/3/p/psi_m;
      | end
      | phi_m_unit = 'V*s';
      | ubez_unit = 'V';
      | ibez_unit = 'A';
      | omega_bez_unit = 'rad/s';
      | 
      | motor = [gcb, '/pmsm_dq2'];
      | 
      | set_param([motor],'emf_nom','ubez');
      | set_param([motor],'emf_nom_unit',ubez_unit);
      | set_param([motor],'i_nom','ibez');
      | set_param([motor],'i_nom_unit',ibez_unit);
      | set_param([motor],'omega_nom','omega_bez');
      | set_param([motor],'omega_nom_unit',omega_bez_unit);
      | set_param([motor],'poles','poles');
      | set_param([motor],'poles_unit',poles_unit);
      | set_param([motor],'Rs','Rs');
      | set_param([motor],'Rs_unit',Rs_unit);
      | set_param([motor],'Ld','Ld');
      | set_param([motor],'Ld_unit',Ld_unit);
      | set_param([motor],'Lq','Lq');
      | set_param([motor],'Lq_unit',Lq_unit);
      | set_param([motor],'phi_m','phi_m');
      | set_param([motor],'phi_m_unit',phi_m_unit);
      | set_param([motor],'J','J');
      | set_param([motor],'J_unit',J_unit);
      | set_param([motor],'b','b');
      | set_param([motor],'b_unit',b_unit);
      | 
      | controller = [gcb, '/pmsm dq controller'];
      | set_param([controller],'emf_nom','ubez');
      | set_param([controller],'emf_nom_unit',ubez_unit);
      | set_param([controller],'i_nom','ibez');
      | set_param([controller],'i_nom_unit',ibez_unit);
      | set_param([controller],'omega_m_nom','omega_bez');
      | set_param([controller],'omega_m_nom_unit',omega_bez_unit);
      | set_param([controller],'poles','poles');
      | set_param([controller],'Rs','Rs');
      | set_param([controller],'Rs_unit',Rs_unit);
      | set_param([controller],'Ld','Ld');
      | set_param([controller],'Ld_unit',Ld_unit);
      | set_param([controller],'Lq','Lq');
      | set_param([controller],'Lq_unit',Lq_unit);
      | set_param([controller],'phi_m','phi_m');
      | set_param([controller],'phi_m_unit',phi_m_unit);
      | set_param([controller],'kp_w','kp_w');
      | set_param([controller],'ki_w','ki_w');
      | set_param([controller],'kp_i','kp_i');
      | set_param([controller],'ki_i','ki_i');
      | set_param([controller],'kp_fw','kp_fw');
      | set_param([controller],'ki_fw','ki_fw');
      | switch cm
      |     case 'Speed Mode'
      |         set_param([controller],'Speed_mode','simscape.enum.onoff.on');
      |     case 'Torque Mode'
      |         set_param([controller],'Speed_mode','simscape.enum.onoff.off');
      | end
      | switch tl
      |     case 'Torque limited from torque ref'
      |         set_param([controller],'TorqueLim','simscape.enum.onoff.on');
      |     case 'Torque unlimited'
      |         set_param([controller],'TorqueLim','simscape.enum.onoff.off');
      | end
      mask Help: eval('open \documentation\pmsm_ctrl_i.pdf')
      mask TypeOptions control_mode: Speed Mode | Torque Mode
      mask TypeOptions torque_limitation: Torque limited from torque ref | Torque unlimited
      mask TypeOptions poles_unit: 1
      mask TypeOptions omega_m_max_unit: rpm
      mask TypeOptions omega_m_nom_unit: rpm
      mask TypeOptions tau_nom_unit: N*m
      mask TypeOptions Rs_unit: Ohm
      mask TypeOptions Ld_unit: H
      mask TypeOptions Lq_unit: H
      mask TypeOptions Ke_unit: V*s
      mask TypeOptions Kt_unit: N*m/Arms
      mask TypeOptions J_unit: kg*m^2
      mask TypeOptions b_unit: N*m/(rad/s)
      mask DialogControl ModeofOperation Prompt: Mode of Operation
      mask DialogControl MotorParameters Prompt: Motor Parameters
      mask DialogControl ControlParameters Prompt: Control Parameters
      mask Display:
      | % Icon = 'C:\Users\dbagn\Dropbox\davide\11_matlab\11.73 HydraulicComponents\IM.jpg'
      | 
      | 
      | modelname = [gcb];
      | % image(imread("library\+pmsm_dq2\pmsm_drawing_mask.png"));
      | 
      | color('red')
      | port_label('lconn',1,'Speed Reference');
      | color('red')
      | port_label('lconn',2,'Maximum Torque');
      | color('blue')
      | port_label('lconn',3,'Uin+');
      | color('blue')
      | port_label('lconn',4,'Uin-');
      | color('black')
      | port_label('output',1,'PMSM data');
      | color('green')
      | port_label('rconn',1,'D')
  shaft : PMIOPort  Side=Right
  Uin+ : PMIOPort  Port=2  Side=Left
  Uin- : PMIOPort  Port=3  Side=Left
  PMSM_Data : Outport
  wires:
  Transfer Fcn6/1 -> Gain/1
  Step1/1 -> Rate Limiter1/1
  Rate Limiter1/1 -> Transfer Fcn6/1
  pmsm_dq_ctrl/1(Data) -> Selector/1, PMSM_Data/1
  Gain/1 -> Sum/1
  Rate Limiter2/1 -> Transfer Fcn1/1
  Step2/1 -> Rate Limiter2/1
  Sum/1 -> Simulink-PS Converter/1
  Transfer Fcn1/1 -> Gain1/1
  Gain1/1 -> Sum/2
  Selector/1 -> Demux/1
  Demux/1 -> Magnitude Squared/1
  Demux/2 -> Magnitude Squared1/1
  Magnitude Squared/1 -> Sum1/1
  Magnitude Squared1/1 -> Sum1/2
  Sum1/1 -> Sqrt/1
  Sqrt/1 -> Gain2/1
  PS-Simulink Converter11/1 -> Scope/2  "udc"
  Gain2/1 -> Scope/1  "ug"
  connections:
  Mechanical Rotational Reference2/LConn1 -- Ideal Torque Source/RConn2
  Ideal Torque Source/LConn1 -- shaft/RConn1 -- flexible shaft/RConn1
  Simulink-PS Converter/RConn1 -- Ideal Torque Source/RConn1
  flexible shaft/LConn1 -- pmsm_dq_ctrl/RConn1
  Voltage Sensor/LConn1 -- pmsm_dq_ctrl/LConn3 -- Uin+/RConn1
  Voltage Sensor/RConn2 -- pmsm_dq_ctrl/LConn4 -- Uin-/RConn1
  Voltage Sensor/RConn1 -- PS-Simulink Converter11/LConn1
  pmsm_dq_ctrl/LConn1 -- PS Constant2/RConn1
  pmsm_dq_ctrl/LConn2 -- PS Constant3/RConn1

== system hdv_hydroelectropowertrain_model/PR776_powertrain/front_blade_model/blade_height ==
  Rate Limiter : RateLimiter  RisingSlewLimit=0.02  FallingSlewLimit=-0.02  SampleTimeMode=inherited
  Saturation : Saturate  UpperLimit=1  LowerLimit=0
  Step5 : Step  Time=simulation_length/3  After=0.5  SampleTime=0
  Transfer Fcn : TransferFcn  Denominator=[1e-2 1]
  blade_height : Outport
  wires:
  Saturation/1 -> Transfer Fcn/1
  Transfer Fcn/1 -> blade_height/1
  Rate Limiter/1 -> Saturation/1
  Step5/1 -> Rate Limiter/1

== system hdv_hydroelectropowertrain_model/PR776_powertrain/front_blade_model/hose ==
  Constant Area Hydraulic Orifice : fl_lib/Hydraulic/Hydraulic Elements/Constant Area Hydraulic Orifice  area=1e-8 m^2  C_d=0.7  lam_spec=1  B_lam=0.999  Re_cr=12  q_specify=off  q_priority=None  q=0.001 m^3/s  q_nominal_specify=off  q_nominal_unit=m^3/s  q_nominal_value=1  p_specify=off  p_priority=None  p=0 Pa  p_nominal_specify=off  p_nominal_unit=Pa  p_nominal_value=1
      settings: InternalSimscapePortConfiguration="{\"Bottom\":[],\"Left\":[{\"id\":\"A\",\"label\":\"A\",\"type\":\"foundation.hydraulic.hydraulic\"}],\"Right\":[{\"id\":\"B\",\"label\":\"B\",\"type\":\"foundation.hydraulic.hydraulic\"}],\"Top\":[]}"
  Constant Area Hydraulic Orifice1 : fl_lib/Hydraulic/Hydraulic Elements/Constant Area Hydraulic Orifice  area=1e-8 m^2  C_d=0.7  lam_spec=1  B_lam=0.999  Re_cr=12  q_specify=off  q_priority=None  q=0.001 m^3/s  q_nominal_specify=off  q_nominal_unit=m^3/s  q_nominal_value=1  p_specify=off  p_priority=None  p=0 Pa  p_nominal_specify=off  p_nominal_unit=Pa  p_nominal_value=1
      settings: InternalSimscapePortConfiguration="{\"Bottom\":[],\"Left\":[{\"id\":\"A\",\"label\":\"A\",\"type\":\"foundation.hydraulic.hydraulic\"}],\"Right\":[{\"id\":\"B\",\"label\":\"B\",\"type\":\"foundation.hydraulic.hydraulic\"}],\"Top\":[]}"
  Hydraulic Flow Rate Sensor3 : fl_lib/Hydraulic/Hydraulic Sensors/Hydraulic Flow Rate Sensor
  Hydraulic Flow Rate Source : fl_lib/Hydraulic/Hydraulic Sources/Hydraulic Flow Rate Source
      settings: InternalSimscapePortConfiguration="{\"Bottom\":[],\"Left\":[{\"id\":\"P\",\"label\":\"P\",\"type\":\"foundation.hydraulic.hydraulic\"}],\"Right\":[{\"id\":\"S\",\"label\":\"S\",\"type\":\"input\"},{\"id\":\"T\",\"label\":\"T\",\"type\":\"foundation.hydraulic.hydraulic\"}],\"Top\":[]}"
  Hydraulic Pressure Sensor2 : fl_lib/Hydraulic/Hydraulic Sensors/Hydraulic Pressure Sensor
  Hydraulic Pressure Source : fl_lib/Hydraulic/Hydraulic Sources/Hydraulic Pressure Source
      settings: InternalSimscapePortConfiguration="{\"Bottom\":[],\"Left\":[{\"id\":\"P\",\"label\":\"P\",\"type\":\"foundation.hydraulic.hydraulic\"}],\"Right\":[{\"id\":\"S\",\"label\":\"S\",\"type\":\"input\"},{\"id\":\"T\",\"label\":\"T\",\"type\":\"foundation.hydraulic.hydraulic\"}],\"Top\":[]}"
  Hydraulic Reference : fl_lib/Hydraulic/Hydraulic Elements/Hydraulic Reference
  PS Gain : fl_lib/Physical Signals/Functions/PS Gain  gain=1 Pa
  PS Gain1 : fl_lib/Physical Signals/Functions/PS Gain  gain=1 Pa^-1
  PS Gain2 : fl_lib/Physical Signals/Functions/PS Gain  gain=1 m^3/s
  PS Gain3 : fl_lib/Physical Signals/Functions/PS Gain  gain=1 m^-3*s
  PS Transfer Function : fl_lib/Physical Signals/Linear Operators/PS Transfer Function  transfer_function_type=foundation.enum.transfer_function_type.lag  T=0.1 s  T1=2 s  T2=1 s  reset_method=foundation.enum.IntegratorResetSpec.None  initial_condition_spec=foundation.enum.IntegratorICSpec.Internal  y0=0
      settings: InternalSimscapePortConfiguration="{\"Bottom\":[],\"Left\":[{\"id\":\"U\",\"label\":\"\",\"type\":\"input\"}],\"Right\":[{\"id\":\"Y\",\"label\":\"\",\"type\":\"output\"}],\"Top\":[]}"
  PS Transfer Function1 : fl_lib/Physical Signals/Linear Operators/PS Transfer Function  transfer_function_type=foundation.enum.transfer_function_type.lag  T=0.1 s  T1=2 s  T2=1 s  reset_method=foundation.enum.IntegratorResetSpec.None  initial_condition_spec=foundation.enum.IntegratorICSpec.Internal  y0=0
      settings: InternalSimscapePortConfiguration="{\"Bottom\":[],\"Left\":[{\"id\":\"U\",\"label\":\"\",\"type\":\"input\"}],\"Right\":[{\"id\":\"Y\",\"label\":\"\",\"type\":\"output\"}],\"Top\":[]}"
  A : PMIOPort  Side=Left
  ps : PMIOPort  Port=2  Side=Right
  B : PMIOPort  Port=3  Side=Left
  pt : PMIOPort  Port=4  Side=Right
  connections:
  ps/RConn1 -- Constant Area Hydraulic Orifice1/LConn1 -- Hydraulic Flow Rate Sensor3/RConn2
  PS Gain2/RConn1 -- Hydraulic Flow Rate Source/RConn1
  Hydraulic Flow Rate Sensor3/RConn1 -- PS Gain3/LConn1
  Hydraulic Flow Rate Sensor3/LConn1 -- Hydraulic Pressure Source/LConn1
  Hydraulic Pressure Source/RConn1 -- PS Gain/RConn1
  PS Gain1/LConn1 -- Hydraulic Pressure Sensor2/RConn2
  Hydraulic Pressure Source/RConn2 -- Hydraulic Pressure Sensor2/RConn1 -- Constant Area Hydraulic Orifice/RConn1 -- B/RConn1 -- Hydraulic Flow Rate Source/LConn1 -- Constant Area Hydraulic Orifice1/RConn1 -- Hydraulic Reference/LConn1 -- pt/RConn1
  PS Transfer Function1/RConn1 -- PS Gain2/LConn1
  PS Transfer Function/RConn1 -- PS Gain/LConn1
  A/RConn1 -- Constant Area Hydraulic Orifice/LConn1 -- Hydraulic Pressure Sensor2/LConn1 -- Hydraulic Flow Rate Source/RConn2
  PS Gain3/RConn1 -- PS Transfer Function1/LConn1
  PS Gain1/RConn1 -- PS Transfer Function/LConn1

== system hdv_hydroelectropowertrain_model/PR776_powertrain/front_blade_model/piston_tilt ==
  ref : Inport
  PS-Simulink Converter{1..5,7,9} (7 alike) : nesl_utility/PS-Simulink Converter  PhysicalDomain=network_engine_domain  SubClassName=ps_output  LeftPortType=input  RightPortType=output  PseudoPeriodic=off  Frequencies=[]  VectorFormat=1-D array  Unit=inherit  AffineConversion=off
  bichamber piston A : bichamber_piston_lib/bichamber piston  A1=8e-3 m^2  A2=8e-3 m^2  Lp=1 m  mp=35 kg  kp=0 N/m  bp=1e3 N/(m/s)  V0=12 l  q1_specify=off  q1_priority=None  q1=0 m^3/s  q1_nominal_specify=off  q1_nominal_unit=m^3/s  q1_nominal_value=1  q2_specify=off  q2_priority=None  q2=0 m^3/s  q2_nominal_specify=off  q2_nominal_unit=m^3/s  q2_nominal_value=1  p1_specify=off  p1_priority=High  p1=0 bar  p1_nominal_specify=off  p1_nominal_unit=bar  p1_nominal_value=1  p2_specify=off  p2_priority=High  p2=0 bar  p2_nominal_specify=off  p2_nominal_unit=bar  p2_nominal_value=1  fp_specify=off  fp_priority=None  fp=0 N  fp_nominal_specify=off  fp_nominal_unit=N  fp_nominal_value=1  vp_specify=off  vp_priority=None  vp=0 m/s  vp_nominal_specify=off  vp_nominal_unit=m/s  vp_nominal_value=1  xp_specify=off  xp_priority=High  xp=0 m  xp_nominal_specify=off  xp_nominal_unit=m  xp_nominal_value=1
      settings: InternalSimscapePortConfiguration="{\"Bottom\":[],\"Left\":[{\"id\":\"H1\",\"label\":\"H1\",\"type\":\"foundation.hydraulic.hydraulic\"},{\"id\":\"H2\",\"label\":\"H2\",\"type\":\"foundation.hydraulic.hydraulic\"}],\"Right\":[{\"id\":\"P\",\"label\":\"P\",\"type\":\"foundation.mechanical.translational.translational\"},{\"id\":\"xp_out\",\"label\":\"xp\",\"type\":\"output\"},{\"id\":\"vp_out\",\"label\":\"vp\",\"type\":\"output\"},{\"id\":\"mforce\",\"label\":\"fm\",\"type\":\"output\"},{\"id\":\"q1_out\",\"label\":\"q1\",\"type\":\"output\"},{\"id\":\"q2_out\",\"label\":\"q2\",\"type\":\"output\"},{\"id\":\"p1_out\",\"label\":\"p1\",\"type\":\"output\"},{\"id\":\"p2_out\",\"label\":\"p2\",\"type\":\"output\"}],\"Top\":[]}"
  blade_tilt_model : Subsystem
  controller : Subsystem
  flow : Scope  NumInputPorts=2
  fm : Scope
  fourway_threeland_valve : fourway_threeland_valve_lib/fourway_threeland_valve  xv_max=valve_mmorifice_max mm  q1_specify=off  q1_priority=None  q1=0 m^3/s  q1_nominal_specify=off  q1_nominal_unit=m^3/s  q1_nominal_value=1  q2_specify=off  q2_priority=None  q2=0 m^3/s  q2_nominal_specify=off  q2_nominal_unit=m^3/s  q2_nominal_value=1  qin_specify=off  qin_priority=None  qin=0 m^3/s  qin_nominal_specify=off  qin_nominal_unit=m^3/s  qin_nominal_value=1  qout_specify=off  qout_priority=None  qout=0 m^3/s  qout_nominal_specify=off  qout_nominal_unit=m^3/s  qout_nominal_value=1  p1_specify=off  p1_priority=None  p1=0 bar  p1_nominal_specify=off  p1_nominal_unit=bar  p1_nominal_value=1  p2_specify=off  p2_priority=None  p2=0 bar  p2_nominal_specify=off  p2_nominal_unit=bar  p2_nominal_value=1  ps_specify=off  ps_priority=None  ps=0 bar  ps_nominal_specify=off  ps_nominal_unit=bar  ps_nominal_value=1  pt_specify=off  pt_priority=None  pt=0 bar  pt_nominal_specify=off  pt_nominal_unit=bar  pt_nominal_value=1
      settings: InternalSimscapePortConfiguration="{\"Bottom\":[],\"Left\":[{\"id\":\"xv\",\"label\":\"xv\",\"type\":\"input\"},{\"id\":\"S\",\"label\":\"S\",\"type\":\"foundation.hydraulic.hydraulic\"},{\"id\":\"T\",\"label\":\"T\",\"type\":\"foundation.hydraulic.hydraulic\"}],\"Right\":[{\"id\":\"H1\",\"label\":\"H1\",\"type\":\"foundation.hydraulic.hydraulic\"},{\"id\":\"H2\",\"label\":\"H2\",\"type\":\"foundation.hydraulic.hydraulic\"}],\"Top\":[]}"
  p1/p2 : Scope  NumInputPorts=2
  xp/vp : Scope  NumInputPorts=2
  xp_re/xp : Scope  NumInputPorts=2
  ps : PMIOPort  Side=Left
  pt : PMIOPort  Port=2  Side=Left
  load : PMIOPort  Port=3  Side=Right
  wires:
  ref/1 -> blade_tilt_model/1(xp_ref), xp_re/xp/1, controller/1(ref)
  PS-Simulink Converter3/1 -> p1/p2/1  "p1"
  PS-Simulink Converter7/1 -> controller/2(xp), xp_re/xp/2, xp/vp/1  "xp"
  PS-Simulink Converter4/1 -> flow/2  "q2"
  PS-Simulink Converter9/1 -> xp/vp/2  "vp"
  PS-Simulink Converter5/1 -> p1/p2/2  "p2"
  PS-Simulink Converter1/1 -> flow/1  "q1"
  PS-Simulink Converter2/1 -> fm/1  "fm"
  connections:
  bichamber piston A/RConn3 -- PS-Simulink Converter9/LConn1
  bichamber piston A/LConn2 -- fourway_threeland_valve/RConn2
  bichamber piston A/LConn1 -- fourway_threeland_valve/RConn1
  bichamber piston A/RConn2 -- PS-Simulink Converter7/LConn1
  bichamber piston A/RConn4 -- PS-Simulink Converter2/LConn1
  bichamber piston A/RConn5 -- PS-Simulink Converter1/LConn1
  bichamber piston A/RConn6 -- PS-Simulink Converter4/LConn1
  bichamber piston A/RConn7 -- PS-Simulink Converter3/LConn1
  bichamber piston A/RConn8 -- PS-Simulink Converter5/LConn1
  ps/RConn1 -- fourway_threeland_valve/LConn2
  pt/RConn1 -- fourway_threeland_valve/LConn3
  fourway_threeland_valve/LConn1 -- controller/RConn1
  blade_tilt_model/LConn1 -- bichamber piston A/RConn1
  load/RConn1 -- blade_tilt_model/RConn1
